simulink model "eVTOL_System"  (R2024b)
settings: Solver=FixedStepAuto  StartTime=0.0  StopTime=inf  RelTol=1e-3
undefined symbols (not defined in the file): airspeed, Battery, BCE12, BCE_Set_init, BMS_Controller_State, C, Cell10_P, Cell11_P, Cell12_P, Cell13_P, Cell14_P, Cell15_P, Cell16_P, Cell17_P, Cell18_P, Cell19_P, Cell1_N, Cell1_P, Cell20_P, Cell21_P, Cell22_P, Cell23_P, Cell24_P, Cell2_P, Cell3_P, Cell4_P, Cell5_P, Cell6_P, Cell7_P, Cell8_P, Cell9_P, Charging_State, CityMission, control, controlParams, ControlSampleTime, CriticalTiltAngle, currentFactor, CV_Gain, ddx, ddy, ddz, Device_01, Device_02, DiscIntNeverNeededParam, dx, dy, dz, Earth, env, F, F28379D_ADC_MaxCount, F28379D_ADC_Vmax, FixedWingMission, flightState, Foc_Ki_IxTcpu, Foc_Ki_S, Foc_Kp_I, Foc_Kp_S, fractalcoef ... (+68)
libraries: fl_lib x1115, nesl_utility x617, slrealtimeethercatlib x217, simulink x130, canmsglib x101, speedgoatlib_IO611_obsolete x91, slpidlib x49, mcbcontrolslib x44, slrealtimeutilitieslib x35, speedgoatlib_hdlCoder_IO3xx x31, dspstat3 x24, mcbpositiondecoderlib x12
(part 24 of 31)

== system eVTOL_System/Flight Controller/Guidance Test Bench/ControlType/Guidance Testbench/Guidance Logic/Guidance Stateflow/Guidance Mode Selector/GuidanceLogic.FIXED_WING_ORBIT.ORBIT ==
  ToWP : Inport
  States : Inport  Port=2
  Action Port : ActionPort
      settings: CopyFcn=Stateflow.SLINSF.SimulinkMan.removeBlockPreDeleteFcn  PreDeleteFcn=Stateflow.SLINSF.SimulinkMan.unsafePredeleteFcn
  Abs1 : Abs  SaturateOnIntegerOverflow=off
  Bus Creator : BusCreator  Inputs=5  OutDataTypeStr=Bus: AAC  NonVirtualBus=on
      settings: InheritFromInputs=off
  Bus Selector : BusSelector  OutputSignals=position,params
  Bus Selector1 : BusSelector  OutputSignals=Xe,course  OutputAsBus=on
  Bus to Vector : BusToVector
  Constant : Constant  Value=control.cruiseSpeed
  Constant1 : Constant  Value=0
  Data Type Conversion : DataTypeConversion  OutDataTypeStr=uint8  SaturateOnIntegerOverflow=off  RndMeth=Floor
  Lookahead Distance : Constant  Value=control.L1  OutDataTypeStr=double
  Relational Operator : RelationalOperator  Operator=>  OutDataTypeStr=boolean  RndMeth=Simplest  InputSameDT=off
  Selector : Selector  InputPortWidth=3  IndexOptions=Index vector (dialog)  Indices=3  OutputSizes=1
  Selector1 : Selector  InputPortWidth=4  IndexOptions=Index vector (dialog)  Indices=2  OutputSizes=1
  Selector2 : Selector  InputPortWidth=4  IndexOptions=Index vector (dialog)  Indices=1  OutputSizes=1
  Selector3 : Selector  InputPortWidth=4  IndexOptions=Index vector (dialog)  Indices=3  OutputSizes=1
  Terminator{,1..3} (4 alike) : Terminator
  UAV Orbit Follower : uavalgslib/Orbit Follower  UAVType=fixed-wing  MinOrbitRadius=control.turningRadius  MinLookaheadDistance=control.L1  ExternalReset=none  ShowCrossTrackErrorOutput=off  ShowNumTurnsOutput=on  SimulateUsing=Code generation
  Unary Minus : UnaryMinus
  Status : Outport
  aacSP : Outport  Port=2
  wires:
  Bus to Vector/1 -> UAV Orbit Follower/1
  Selector2/1 -> UAV Orbit Follower/3
  Bus Selector/1 -> UAV Orbit Follower/2, Selector/1  "<position>"
  ToWP/1 -> Bus Selector/1
  Bus Selector/2 -> Selector1/1, Selector3/1, Selector2/1  "<params>"
  Selector3/1 -> Relational Operator/2
  Relational Operator/1 -> Data Type Conversion/1
  UAV Orbit Follower/4 -> Terminator/1
  UAV Orbit Follower/5 -> Terminator1/1
  Bus Selector1/1 -> Bus to Vector/1
  States/1 -> Bus Selector1/1
  UAV Orbit Follower/1 -> Terminator2/1  "LAP"
  Lookahead Distance/1 -> UAV Orbit Follower/5, Bus Creator/4  "L1"
  Bus Creator/1 -> aacSP/1
  UAV Orbit Follower/2 -> Bus Creator/3  "course"
  Constant/1 -> Bus Creator/1  "airspeed"
  Unary Minus/1 -> Bus Creator/2  "altitude"
  UAV Orbit Follower/3 -> Terminator3/1  "YawCmd"
  Selector/1 -> Unary Minus/1
  UAV Orbit Follower/6 -> Abs1/1
  Abs1/1 -> Relational Operator/1
  Selector1/1 -> UAV Orbit Follower/4
  Constant1/1 -> Bus Creator/5  "climbrate"
  Data Type Conversion/1 -> Status/1

== system eVTOL_System/Flight Controller/Guidance Test Bench/ControlType/Guidance Testbench/Guidance Logic/Guidance Stateflow/Guidance Mode Selector/GuidanceLogic.FIXED_WING_WAYPOINT.WAYPOINT ==
  note: This subsystem selects a lookahead point on the path and provides a desired course. Desired course is later converted to desired lateral acceleration (and roll setpoint)
  States : Inport
  ToWP : Inport  Port=2
  FromWP : Inport  Port=3
  Action Port : ActionPort
      settings: CopyFcn=Stateflow.SLINSF.SimulinkMan.removeBlockPreDeleteFcn  PreDeleteFcn=Stateflow.SLINSF.SimulinkMan.unsafePredeleteFcn
  Bus Creator : BusCreator  Inputs=5  OutDataTypeStr=Bus: AAC  NonVirtualBus=on
      settings: InheritFromInputs=off
  Bus Selector : BusSelector  OutputSignals=Xe,course  OutputAsBus=on
  Bus Selector1 : BusSelector  OutputSignals=position
  Bus Selector2 : BusSelector  OutputSignals=position
  Bus to Vector : BusToVector
  Constant : Constant  Value=control.cruiseSpeed
  Constant1 : Constant  Value=0
  Data Type Conversion : DataTypeConversion  SaturateOnIntegerOverflow=off  RndMeth=Floor
  Lookahead Distance : Constant  Value=control.L1  OutDataTypeStr=double
  MATLAB Function : MATLAB Function  TreatAsAtomicUnit=on
  Scope : Scope
  Terminator : Terminator
  Terminator1 : Terminator
  Terminator2 : Terminator
  Waypoint Follower : uavalgslib/Waypoint Follower  UAVType=fixed-wing  StartFrom=first  TransitionRadiusSource=internal  TransitionRadius=FWControl.transitionRadius  MinLookaheadDistance=control.L1  HoverAtLastWaypoint=off  YawInput=off  ShowCrossTrackErrorOutput=off  ShowStatusOutput=on  SimulateUsing=Code generation
  Status : Outport
  aacSP : Outport  Port=2
  wires:
  Lookahead Distance/1 -> Waypoint Follower/3, Bus Creator/4  "L1"
  Waypoint Follower/1 -> Terminator/1  "LAP"
  Waypoint Follower/3 -> Terminator1/1  "YawCmd"
  Waypoint Follower/4 -> Terminator2/1
  Constant/1 -> Bus Creator/1  "airspeed"
  States/1 -> Bus Selector/1
  Bus Selector/1 -> Bus to Vector/1
  Waypoint Follower/5 -> Scope/1, Data Type Conversion/1
  Data Type Conversion/1 -> Status/1
  Bus Creator/1 -> aacSP/1
  MATLAB Function/1(wps) -> Waypoint Follower/2
  Bus to Vector/1 -> Waypoint Follower/1
  ToWP/1 -> Bus Selector1/1
  FromWP/1 -> Bus Selector2/1
  Bus Selector1/1 -> MATLAB Function/1(toWP)  "<position>"
  Bus Selector2/1 -> MATLAB Function/2(fromWP)  "<position>"
  MATLAB Function/2(alt) -> Bus Creator/2
  Waypoint Follower/2 -> Bus Creator/3  "course"
  Constant1/1 -> Bus Creator/5  "climbrate"

== system eVTOL_System/Flight Controller/Guidance Test Bench/ControlType/Guidance Testbench/Guidance Logic/Guidance Stateflow/Guidance Mode Selector/GuidanceLogic.ForwardTransition ==
  Action Port : ActionPort
      settings: CopyFcn=Stateflow.SLINSF.SimulinkMan.removeBlockPreDeleteFcn  PreDeleteFcn=Stateflow.SLINSF.SimulinkMan.unsafePredeleteFcn
  Bus Creator1 : BusCreator  Inputs=3  OutDataTypeStr=Bus: innerLoopCmdsBus  NonVirtualBus=on
  Constant : Constant  Value=0
  Constant1 : Constant  Value=0
  Constant2 : Constant  Value=0
  Constant3 : Constant  Value=[0 0 0]
  Data Type Conversion : DataTypeConversion  OutDataTypeStr=uint8  SaturateOnIntegerOverflow=off  RndMeth=Floor
  Status : Outport
  InnerLoopCmds : Outport  Port=2  OutDataTypeStr=Bus: innerLoopCmdsBus
  wires:
  Constant3/1 -> Bus Creator1/1  "LAP"
  Bus Creator1/1 -> InnerLoopCmds/1
  Constant1/1 -> Bus Creator1/2  "HeadingCmd"
  Constant2/1 -> Bus Creator1/3  "YawCmd"
  Data Type Conversion/1 -> Status/1
  Constant/1 -> Data Type Conversion/1

== system eVTOL_System/Flight Controller/Guidance Test Bench/ControlType/Guidance Testbench/Guidance Logic/Guidance Stateflow/Guidance Mode Selector/GuidanceLogic.Land.Descend ==
  ToWP : Inport
  Action Port : ActionPort
      settings: CopyFcn=Stateflow.SLINSF.SimulinkMan.removeBlockPreDeleteFcn  PreDeleteFcn=Stateflow.SLINSF.SimulinkMan.unsafePredeleteFcn
  Bus Creator : BusCreator  Inputs=3  OutDataTypeStr=Bus: innerLoopCmdsBus  NonVirtualBus=on
      settings: InheritFromInputs=off
  Bus Selector : BusSelector  OutputSignals=position,params
  Demux1 : Demux  Outputs=[2 1]
  Hdg Cmd Sat : Saturate  UpperLimit=pi  LowerLimit=-pi
      settings: AttributesFormatString=[%<UpperLimit> %<LowerLimit>]
  Mux : Mux  Inputs=2
  Selector1 : Selector  InputPortWidth=4  IndexOptions=Index vector (dialog)  Indices=4  OutputSizes=1
  Selector3 : Selector  InputPortWidth=4  IndexOptions=Index vector (dialog)  Indices=4  OutputSizes=1
  Yaw Cmd Sat : Saturate  UpperLimit=pi  LowerLimit=-pi
      settings: AttributesFormatString=[%<UpperLimit> %<LowerLimit>]
  InnerLoopCmds : Outport  OutDataTypeStr=Bus: innerLoopCmdsBus
  wires:
  Bus Creator/1 -> InnerLoopCmds/1
  Mux/1 -> Bus Creator/1  "LAP"
  Bus Selector/2 -> Selector1/1, Selector3/1  "<params>"
  Bus Selector/1 -> Demux1/1  "<position>"
  Yaw Cmd Sat/1 -> Bus Creator/3  "YawCmd"
  Hdg Cmd Sat/1 -> Bus Creator/2  "HeadingCmd"
  ToWP/1 -> Bus Selector/1
  Demux1/2 -> Mux/2
  Demux1/1 -> Mux/1
  Selector1/1 -> Yaw Cmd Sat/1
  Selector3/1 -> Hdg Cmd Sat/1

== system eVTOL_System/Flight Controller/Guidance Test Bench/ControlType/Guidance Testbench/Guidance Logic/Guidance Stateflow/Guidance Mode Selector/GuidanceLogic.Land.ToLand ==
  Pose : Inport
  ToWP : Inport  Port=2
  FromWP : Inport  Port=3
  Action Port : ActionPort
      settings: CopyFcn=Stateflow.SLINSF.SimulinkMan.removeBlockPreDeleteFcn  PreDeleteFcn=Stateflow.SLINSF.SimulinkMan.unsafePredeleteFcn
  Bus Creator1 : BusCreator  Inputs=3  OutDataTypeStr=Bus: innerLoopCmdsBus  NonVirtualBus=on
  Constant : Constant  Value=0  OutDataTypeStr=uint8
  Lookahead Distance : Constant  Value=15  OutDataTypeStr=double
  MATLAB Function : MATLAB Function  TreatAsAtomicUnit=on
  Scope : Scope
  Waypoint Follower : uavalgslib/Waypoint Follower  UAVType=multirotor  StartFrom=closest  TransitionRadiusSource=internal  TransitionRadius=10  MinLookaheadDistance=0.1  HoverAtLastWaypoint=off  YawInput=on  ShowCrossTrackErrorOutput=off  ShowStatusOutput=off  SimulateUsing=Code generation
  Status : Outport
  InnerLoopCmds : Outport  Port=2  OutDataTypeStr=Bus: innerLoopCmdsBus
  wires:
  Constant/1 -> Status/1
  MATLAB Function/1(wps) -> Waypoint Follower/2
  Lookahead Distance/1 -> Waypoint Follower/3
  Bus Creator1/1 -> InnerLoopCmds/1
  ToWP/1 -> MATLAB Function/2(ToWP)
  Waypoint Follower/2 -> Bus Creator1/2  "HeadingCmd"
  FromWP/1 -> MATLAB Function/1(FromWP)
  Waypoint Follower/4 -> Scope/1
  Waypoint Follower/3 -> Bus Creator1/3  "YawCmd"
  Pose/1 -> Waypoint Follower/1
  Waypoint Follower/1 -> Bus Creator1/1  "LAP"

== system eVTOL_System/Flight Controller/Guidance Test Bench/ControlType/Guidance Testbench/Guidance Logic/Guidance Stateflow/Guidance Mode Selector/GuidanceLogic.Land.WingsLevel ==
  Pose : Inport
  ToWP : Inport  Port=2
  FromWP : Inport  Port=3
  Action Port : ActionPort
      settings: CopyFcn=Stateflow.SLINSF.SimulinkMan.removeBlockPreDeleteFcn  PreDeleteFcn=Stateflow.SLINSF.SimulinkMan.unsafePredeleteFcn
  Bus Creator1 : BusCreator  Inputs=3  OutDataTypeStr=Bus: innerLoopCmdsBus  NonVirtualBus=on
  Constant : Constant  Value=0  OutDataTypeStr=uint8
  Constant1 : Constant  Value=0
  Constant2 : Constant  Value=0
  MATLAB Function : MATLAB Function  TreatAsAtomicUnit=on
  Terminator : Terminator
  Status : Outport
  InnerLoopCmds : Outport  Port=2  OutDataTypeStr=Bus: innerLoopCmdsBus
  wires:
  Bus Creator1/1 -> InnerLoopCmds/1
  Constant/1 -> Status/1
  MATLAB Function/1(outWPS) -> Bus Creator1/1  "LAP"
  Constant1/1 -> Bus Creator1/2  "HeadingCmd"
  FromWP/1 -> MATLAB Function/1(FromWP)
  Constant2/1 -> Bus Creator1/3  "YawCmd"
  ToWP/1 -> MATLAB Function/2(ToWP)
  Pose/1 -> Terminator/1

== system eVTOL_System/Flight Controller/Guidance Test Bench/ControlType/Guidance Testbench/Guidance Logic/Guidance Stateflow/Guidance Mode Selector/GuidanceLogic.Orbit ==
  ToWP : Inport
  Pose : Inport  Port=2
  Action Port : ActionPort
      settings: CopyFcn=Stateflow.SLINSF.SimulinkMan.removeBlockPreDeleteFcn  PreDeleteFcn=Stateflow.SLINSF.SimulinkMan.unsafePredeleteFcn
  Abs : Abs  SaturateOnIntegerOverflow=off
  Bus Creator : BusCreator  Inputs=3  OutDataTypeStr=Bus: innerLoopCmdsBus  NonVirtualBus=on
  Bus Selector : BusSelector  OutputSignals=position,params
  Data Type Conversion : DataTypeConversion  OutDataTypeStr=uint8  SaturateOnIntegerOverflow=off  RndMeth=Floor
  Lookahead Distance : Constant  Value=5  OutDataTypeStr=double
  Radius : Selector  InputPortWidth=4  IndexOptions=Index vector (dialog)  Indices=[3]  OutputSizes=1
  Relational Operator : RelationalOperator  Operator=>  OutDataTypeStr=boolean  RndMeth=Simplest  InputSameDT=off
  Sign : Signum  ZeroCross=off
  Terminator : Terminator
  Terminator1 : Terminator
  Turns : Selector  InputPortWidth=4  IndexOptions=Index vector (dialog)  Indices=[1]  OutputSizes=1
  UAV Orbit Follower : uavalgslib/Orbit Follower  UAVType=multirotor  MinOrbitRadius=1  MinLookaheadDistance=0.1  ExternalReset=none  ShowCrossTrackErrorOutput=off  ShowNumTurnsOutput=on  SimulateUsing=Code generation
  InnerLoopCmds : Outport  OutDataTypeStr=Bus: innerLoopCmdsBus
  Status : Outport  Port=2
  wires:
  Pose/1 -> UAV Orbit Follower/1
  Lookahead Distance/1 -> UAV Orbit Follower/5
  Abs/1 -> UAV Orbit Follower/3
  Bus Selector/1 -> UAV Orbit Follower/2  "<position>"
  ToWP/1 -> Bus Selector/1
  UAV Orbit Follower/1 -> Bus Creator/1  "LAP"
  Bus Creator/1 -> InnerLoopCmds/1
  UAV Orbit Follower/2 -> Bus Creator/2  "HeadingCmd"
  UAV Orbit Follower/3 -> Bus Creator/3  "YawCmd"
  Bus Selector/2 -> Turns/1, Radius/1  "<params>"
  Radius/1 -> Abs/1, Sign/1
  Sign/1 -> UAV Orbit Follower/4
  Relational Operator/1 -> Data Type Conversion/1
  Turns/1 -> Relational Operator/2
  Data Type Conversion/1 -> Status/1
  UAV Orbit Follower/6 -> Relational Operator/1
  UAV Orbit Follower/4 -> Terminator/1
  UAV Orbit Follower/5 -> Terminator1/1

== system eVTOL_System/Flight Controller/Guidance Test Bench/ControlType/Guidance Testbench/Guidance Logic/Guidance Stateflow/Guidance Mode Selector/GuidanceLogic.Takeoff ==
  ToWP : Inport
  Pose : Inport  Port=2
  Action Port : ActionPort
      settings: CopyFcn=Stateflow.SLINSF.SimulinkMan.removeBlockPreDeleteFcn  PreDeleteFcn=Stateflow.SLINSF.SimulinkMan.unsafePredeleteFcn
  Bus Creator : BusCreator  Inputs=3  OutDataTypeStr=Bus: innerLoopCmdsBus  NonVirtualBus=on
      settings: InheritFromInputs=off
  Bus Selector : BusSelector  OutputSignals=position,params
  Constant : Constant  Value=0  OutDataTypeStr=uint8
  Constant1 : Constant  Value=0
  Demux : Demux  Outputs=[2 2]
  Demux1 : Demux  Outputs=[2 1]
  Hdg. Cmd Sat : Saturate  UpperLimit=pi  LowerLimit=-pi
      settings: AttributesFormatString=[%<UpperLimit> %<LowerLimit>]
  Mux : Mux  Inputs=2
  Selector3 : Selector  InputPortWidth=4  IndexOptions=Index vector (dialog)  Indices=4  OutputSizes=1
  Terminator : Terminator
  Terminator1 : Terminator
  Yaw Cmd Sat : Saturate  UpperLimit=pi  LowerLimit=-pi
      settings: AttributesFormatString=[%<UpperLimit> %<LowerLimit>]
  InnerLoopCmds : Outport  OutDataTypeStr=Bus: innerLoopCmdsBus
  Status : Outport  Port=2
  wires:
  Hdg. Cmd Sat/1 -> Bus Creator/2  "HeadingCmd"
  Bus Creator/1 -> InnerLoopCmds/1
  Constant/1 -> Status/1
  Pose/1 -> Demux/1
  Yaw Cmd Sat/1 -> Bus Creator/3  "YawCmd"
  ToWP/1 -> Bus Selector/1
  Bus Selector/2 -> Selector3/1  "<params>"
  Mux/1 -> Bus Creator/1  "LAP"
  Demux/1 -> Mux/1
  Bus Selector/1 -> Demux1/1  "<position>"
  Demux/2 -> Terminator/1
  Demux1/1 -> Terminator1/1
  Selector3/1 -> Hdg. Cmd Sat/1
  Constant1/1 -> Yaw Cmd Sat/1
  Demux1/2 -> Mux/2

== system eVTOL_System/Flight Controller/Guidance Test Bench/ControlType/Guidance Testbench/Guidance Logic/Guidance Stateflow/Guidance Mode Selector/GuidanceLogic.WP ==
  FromWP : Inport
  Pose : Inport  Port=2
  ToWP : Inport  Port=3
  Action Port : ActionPort
      settings: CopyFcn=Stateflow.SLINSF.SimulinkMan.removeBlockPreDeleteFcn  PreDeleteFcn=Stateflow.SLINSF.SimulinkMan.unsafePredeleteFcn
  Back Transition Guard : Subsystem
  Bus Creator : BusCreator  Inputs=3  OutDataTypeStr=Bus: innerLoopCmdsBus  NonVirtualBus=on
  Constant : Constant  Value=0
  Data Type Conversion : DataTypeConversion  OutDataTypeStr=uint8  SaturateOnIntegerOverflow=off  RndMeth=Floor
  Dist2WP : Subsystem
  Lookahead Distance : Constant  Value=R_LOOKAHEAD  OutDataTypeStr=double
  MATLAB Function : MATLAB Function  TreatAsAtomicUnit=on
  Relational Operator : RelationalOperator  OutDataTypeStr=boolean  RndMeth=Simplest  InputSameDT=off
  Scope : Scope
  Terminator : Terminator
  Waypoint Follower : uavalgslib/Waypoint Follower  UAVType=multirotor  StartFrom=closest  TransitionRadiusSource=internal  TransitionRadius=R_WAYPOINTTRANSITION  MinLookaheadDistance=0.1  HoverAtLastWaypoint=off  YawInput=on  ShowCrossTrackErrorOutput=off  ShowStatusOutput=off  SimulateUsing=Code generation
  InnerLoopCmds : Outport  OutDataTypeStr=Bus: innerLoopCmdsBus
  Status : Outport  Port=2
  wires:
  Data Type Conversion/1 -> Status/1
  Bus Creator/1 -> InnerLoopCmds/1
  ToWP/1 -> Dist2WP/3(ToWP), MATLAB Function/2(ToWP)
  Waypoint Follower/1 -> Bus Creator/1  "LAP"
  MATLAB Function/1(wps) -> Waypoint Follower/2
  Waypoint Follower/2 -> Bus Creator/2  "HeadingCmd"
  Waypoint Follower/4 -> Scope/1
  Dist2WP/1(Dist) -> Relational Operator/2
  FromWP/1 -> Back Transition Guard/2(FromWP)
  Relational Operator/1 -> Data Type Conversion/1
  Back Transition Guard/1(PrevWP) -> Dist2WP/2(FromWP), MATLAB Function/1(FromWP)
  Pose/1 -> Back Transition Guard/1(Poses), Waypoint Follower/1, Dist2WP/1(Pose)
  Lookahead Distance/1 -> Relational Operator/1, Waypoint Follower/3
  Constant/1 -> Bus Creator/3  "YawCmd"
  Waypoint Follower/3 -> Terminator/1  "YawCmd"

== system eVTOL_System/Motor Drive/Controller/Controller_MIL/F28379D Firmware/Controller Algorithm/FOC/Current Control ==
  Iab : Inport
  Pos : Inport  Port=2
  Enable : Inport  Port=3
  Idq_ref_PU : Inport  Port=4
  SpeedRef : Inport  Port=5
  Kp_i : Inport  Port=6
  Ki_ixTcpu : Inport  Port=7
  Control_System : Subsystem
  ModWave : Outport  InitialOutput=0  VectorParamsAs1DForOutWhenUnconnected=off
  PWM_Enable : Outport  Port=2  InitialOutput=0  VectorParamsAs1DForOutWhenUnconnected=off
  wires:
  Idq_ref_PU/1 -> Control_System/4(Idq_ref_PU)  "Idq_ref"
  Pos/1 -> Control_System/2(Pos_PU)  "Pos_PU"
  Enable/1 -> Control_System/3(Enable)
  Iab/1 -> Control_System/1(Iab_meas_PU)  "Iab"
  SpeedRef/1 -> Control_System/5(SpeedRef)
  Control_System/1(ModWave) -> ModWave/1
  Control_System/2(PWM_Enable) -> PWM_Enable/1
  Kp_i/1 -> Control_System/6(Kp_i)
  Ki_ixTcpu/1 -> Control_System/7(Ki_ixTcpu)

== system eVTOL_System/Motor Drive/Controller/Controller_MIL/F28379D Firmware/Controller Algorithm/FOC/Speed Control MLD ==
  En_closedloop : Inport
  EnablePWM : Inport  Port=2
  SpeedRef : Inport  Port=3
  Speed_Meas_PU : Inport  Port=4
  Kp_S : Inport  Port=5
  Ki_S : Inport  Port=6
  AND : Logic  IconShape=distinctive  AllPortsSameDT=off  OutDataTypeStr=boolean
  Id_Ref : Constant  Value=0  OutDataTypeStr=single
  Mux : Mux  Inputs=2
  PI_Controller_Speed : Subsystem
  Speed_Ref_Selector : Subsystem
  IdqRef_PU : Outport  VectorParamsAs1DForOutWhenUnconnected=off
  wires:
  En_closedloop/1 -> PI_Controller_Speed/1(Enable), AND/1
  EnablePWM/1 -> AND/2
  SpeedRef/1 -> Speed_Ref_Selector/2(SpeedCommand)
  AND/1 -> Speed_Ref_Selector/1(Enable)
  Speed_Meas_PU/1 -> PI_Controller_Speed/3(N_fb), Speed_Ref_Selector/3(Speed_Ref_Open)
  Kp_S/1 -> PI_Controller_Speed/4(Kp_S)
  Speed_Ref_Selector/1(Speed_Ref_PU) -> PI_Controller_Speed/2(N_ref)
  Ki_S/1 -> PI_Controller_Speed/5(Ki_S)
  Id_Ref/1 -> Mux/1
  PI_Controller_Speed/1(Iq_ref) -> Mux/2
  Mux/1 -> IdqRef_PU/1

== system eVTOL_System/Motor Drive/Controller/Controller_MIL/F28379D Firmware/Controller Algorithm/Speed and Pos Decoder/IndexFinder ==
  In1 : Inport
  Enable : EnablePort
  AND : Logic  AllPortsSameDT=off  OutDataTypeStr=boolean
  Compare To Constant : simulink/Logic and Bit Operations/Compare To Constant  relop===  const=0  OutDataTypeStr=boolean
  Compare To Constant1 : simulink/Logic and Bit Operations/Compare To Constant  relop=>  const=0  OutDataTypeStr=boolean
  Delay3 : Delay  DelayLength=1
  IndexFound : Outport
  wires:
  In1/1 -> Delay3/1, Compare To Constant1/1
  Compare To Constant1/1 -> AND/2
  Compare To Constant/1 -> AND/1
  Delay3/1 -> Compare To Constant/1
  AND/1 -> IndexFound/1

== system eVTOL_System/Motor Drive/Controller1/Controller_MIL/F28379D Firmware/Controller Algorithm/FOC/Current Control ==
  Iab : Inport
  Pos : Inport  Port=2
  Enable : Inport  Port=3
  Idq_ref_PU : Inport  Port=4
  SpeedRef : Inport  Port=5
  Kp_i : Inport  Port=6
  Ki_ixTcpu : Inport  Port=7
  Control_System : Subsystem
  ModWave : Outport  InitialOutput=0  VectorParamsAs1DForOutWhenUnconnected=off
  PWM_Enable : Outport  Port=2  InitialOutput=0  VectorParamsAs1DForOutWhenUnconnected=off
  wires:
  Idq_ref_PU/1 -> Control_System/4(Idq_ref_PU)  "Idq_ref"
  Pos/1 -> Control_System/2(Pos_PU)  "Pos_PU"
  Enable/1 -> Control_System/3(Enable)
  Iab/1 -> Control_System/1(Iab_meas_PU)  "Iab"
  SpeedRef/1 -> Control_System/5(SpeedRef)
  Control_System/1(ModWave) -> ModWave/1
  Control_System/2(PWM_Enable) -> PWM_Enable/1
  Kp_i/1 -> Control_System/6(Kp_i)
  Ki_ixTcpu/1 -> Control_System/7(Ki_ixTcpu)

== system eVTOL_System/Motor Drive/Controller1/Controller_MIL/F28379D Firmware/Controller Algorithm/FOC/Speed Control MLD ==
  En_closedloop : Inport
  EnablePWM : Inport  Port=2
  SpeedRef : Inport  Port=3
  Speed_Meas_PU : Inport  Port=4
  Kp_S : Inport  Port=5
  Ki_S : Inport  Port=6
  AND : Logic  IconShape=distinctive  AllPortsSameDT=off  OutDataTypeStr=boolean
  Id_Ref : Constant  Value=0  OutDataTypeStr=single
  Mux : Mux  Inputs=2
  PI_Controller_Speed : Subsystem
  Speed_Ref_Selector : Subsystem
  IdqRef_PU : Outport  VectorParamsAs1DForOutWhenUnconnected=off
  wires:
  En_closedloop/1 -> PI_Controller_Speed/1(Enable), AND/1
  EnablePWM/1 -> AND/2
  SpeedRef/1 -> Speed_Ref_Selector/2(SpeedCommand)
  AND/1 -> Speed_Ref_Selector/1(Enable)
  Speed_Meas_PU/1 -> PI_Controller_Speed/3(N_fb), Speed_Ref_Selector/3(Speed_Ref_Open)
  Kp_S/1 -> PI_Controller_Speed/4(Kp_S)
  Speed_Ref_Selector/1(Speed_Ref_PU) -> PI_Controller_Speed/2(N_ref)
  Ki_S/1 -> PI_Controller_Speed/5(Ki_S)
  Id_Ref/1 -> Mux/1
  PI_Controller_Speed/1(Iq_ref) -> Mux/2
  Mux/1 -> IdqRef_PU/1

== system eVTOL_System/Motor Drive/Controller1/Controller_MIL/F28379D Firmware/Controller Algorithm/Speed and Pos Decoder/IndexFinder ==
  In1 : Inport
  Enable : EnablePort
  AND : Logic  AllPortsSameDT=off  OutDataTypeStr=boolean
  Compare To Constant : simulink/Logic and Bit Operations/Compare To Constant  relop===  const=0  OutDataTypeStr=boolean
  Compare To Constant1 : simulink/Logic and Bit Operations/Compare To Constant  relop=>  const=0  OutDataTypeStr=boolean
  Delay3 : Delay  DelayLength=1
  IndexFound : Outport
  wires:
  In1/1 -> Delay3/1, Compare To Constant1/1
  Compare To Constant1/1 -> AND/2
  Compare To Constant/1 -> AND/1
  Delay3/1 -> Compare To Constant/1
  AND/1 -> IndexFound/1

== system eVTOL_System/Motor Drive/Controller2/Controller_MIL/F28379D Firmware/Controller Algorithm/FOC/Current Control ==
  Iab : Inport
  Pos : Inport  Port=2
  Enable : Inport  Port=3
  Idq_ref_PU : Inport  Port=4
  SpeedRef : Inport  Port=5
  Kp_i : Inport  Port=6
  Ki_ixTcpu : Inport  Port=7
  Control_System : Subsystem
  ModWave : Outport  InitialOutput=0  VectorParamsAs1DForOutWhenUnconnected=off
  PWM_Enable : Outport  Port=2  InitialOutput=0  VectorParamsAs1DForOutWhenUnconnected=off
  wires:
  Idq_ref_PU/1 -> Control_System/4(Idq_ref_PU)  "Idq_ref"
  Pos/1 -> Control_System/2(Pos_PU)  "Pos_PU"
  Enable/1 -> Control_System/3(Enable)
  Iab/1 -> Control_System/1(Iab_meas_PU)  "Iab"
  SpeedRef/1 -> Control_System/5(SpeedRef)
  Control_System/1(ModWave) -> ModWave/1
  Control_System/2(PWM_Enable) -> PWM_Enable/1
  Kp_i/1 -> Control_System/6(Kp_i)
  Ki_ixTcpu/1 -> Control_System/7(Ki_ixTcpu)

== system eVTOL_System/Motor Drive/Controller2/Controller_MIL/F28379D Firmware/Controller Algorithm/FOC/Speed Control MLD ==
  En_closedloop : Inport
  EnablePWM : Inport  Port=2
  SpeedRef : Inport  Port=3
  Speed_Meas_PU : Inport  Port=4
  Kp_S : Inport  Port=5
  Ki_S : Inport  Port=6
  AND : Logic  IconShape=distinctive  AllPortsSameDT=off  OutDataTypeStr=boolean
  Id_Ref : Constant  Value=0  OutDataTypeStr=single
  Mux : Mux  Inputs=2
  PI_Controller_Speed : Subsystem
  Speed_Ref_Selector : Subsystem
  IdqRef_PU : Outport  VectorParamsAs1DForOutWhenUnconnected=off
  wires:
  En_closedloop/1 -> PI_Controller_Speed/1(Enable), AND/1
  EnablePWM/1 -> AND/2
  SpeedRef/1 -> Speed_Ref_Selector/2(SpeedCommand)
  AND/1 -> Speed_Ref_Selector/1(Enable)
  Speed_Meas_PU/1 -> PI_Controller_Speed/3(N_fb), Speed_Ref_Selector/3(Speed_Ref_Open)
  Kp_S/1 -> PI_Controller_Speed/4(Kp_S)
  Speed_Ref_Selector/1(Speed_Ref_PU) -> PI_Controller_Speed/2(N_ref)
  Ki_S/1 -> PI_Controller_Speed/5(Ki_S)
  Id_Ref/1 -> Mux/1
  PI_Controller_Speed/1(Iq_ref) -> Mux/2
  Mux/1 -> IdqRef_PU/1

== system eVTOL_System/Motor Drive/Controller2/Controller_MIL/F28379D Firmware/Controller Algorithm/Speed and Pos Decoder/IndexFinder ==
  In1 : Inport
  Enable : EnablePort
  AND : Logic  AllPortsSameDT=off  OutDataTypeStr=boolean
  Compare To Constant : simulink/Logic and Bit Operations/Compare To Constant  relop===  const=0  OutDataTypeStr=boolean
  Compare To Constant1 : simulink/Logic and Bit Operations/Compare To Constant  relop=>  const=0  OutDataTypeStr=boolean
  Delay3 : Delay  DelayLength=1
  IndexFound : Outport
  wires:
  In1/1 -> Delay3/1, Compare To Constant1/1
  Compare To Constant1/1 -> AND/2
  Compare To Constant/1 -> AND/1
  Delay3/1 -> Compare To Constant/1
  AND/1 -> IndexFound/1

== system eVTOL_System/Motor Drive/Controller3/Controller_MIL/F28379D Firmware/Controller Algorithm/FOC/Current Control ==
  Iab : Inport
  Pos : Inport  Port=2
  Enable : Inport  Port=3
  Idq_ref_PU : Inport  Port=4
  SpeedRef : Inport  Port=5
  Kp_i : Inport  Port=6
  Ki_ixTcpu : Inport  Port=7
  Control_System : Subsystem
  ModWave : Outport  InitialOutput=0  VectorParamsAs1DForOutWhenUnconnected=off
  PWM_Enable : Outport  Port=2  InitialOutput=0  VectorParamsAs1DForOutWhenUnconnected=off
  wires:
  Idq_ref_PU/1 -> Control_System/4(Idq_ref_PU)  "Idq_ref"
  Pos/1 -> Control_System/2(Pos_PU)  "Pos_PU"
  Enable/1 -> Control_System/3(Enable)
  Iab/1 -> Control_System/1(Iab_meas_PU)  "Iab"
  SpeedRef/1 -> Control_System/5(SpeedRef)
  Control_System/1(ModWave) -> ModWave/1
  Control_System/2(PWM_Enable) -> PWM_Enable/1
  Kp_i/1 -> Control_System/6(Kp_i)
  Ki_ixTcpu/1 -> Control_System/7(Ki_ixTcpu)

== system eVTOL_System/Motor Drive/Controller3/Controller_MIL/F28379D Firmware/Controller Algorithm/FOC/Speed Control MLD ==
  En_closedloop : Inport
  EnablePWM : Inport  Port=2
  SpeedRef : Inport  Port=3
  Speed_Meas_PU : Inport  Port=4
  Kp_S : Inport  Port=5
  Ki_S : Inport  Port=6
  AND : Logic  IconShape=distinctive  AllPortsSameDT=off  OutDataTypeStr=boolean
  Id_Ref : Constant  Value=0  OutDataTypeStr=single
  Mux : Mux  Inputs=2
  PI_Controller_Speed : Subsystem
  Speed_Ref_Selector : Subsystem
  IdqRef_PU : Outport  VectorParamsAs1DForOutWhenUnconnected=off
  wires:
  En_closedloop/1 -> PI_Controller_Speed/1(Enable), AND/1
  EnablePWM/1 -> AND/2
  SpeedRef/1 -> Speed_Ref_Selector/2(SpeedCommand)
  AND/1 -> Speed_Ref_Selector/1(Enable)
  Speed_Meas_PU/1 -> PI_Controller_Speed/3(N_fb), Speed_Ref_Selector/3(Speed_Ref_Open)
  Kp_S/1 -> PI_Controller_Speed/4(Kp_S)
  Speed_Ref_Selector/1(Speed_Ref_PU) -> PI_Controller_Speed/2(N_ref)
  Ki_S/1 -> PI_Controller_Speed/5(Ki_S)
  Id_Ref/1 -> Mux/1
  PI_Controller_Speed/1(Iq_ref) -> Mux/2
  Mux/1 -> IdqRef_PU/1

== system eVTOL_System/Motor Drive/Controller3/Controller_MIL/F28379D Firmware/Controller Algorithm/Speed and Pos Decoder/IndexFinder ==
  In1 : Inport
  Enable : EnablePort
  AND : Logic  AllPortsSameDT=off  OutDataTypeStr=boolean
  Compare To Constant : simulink/Logic and Bit Operations/Compare To Constant  relop===  const=0  OutDataTypeStr=boolean
  Compare To Constant1 : simulink/Logic and Bit Operations/Compare To Constant  relop=>  const=0  OutDataTypeStr=boolean
  Delay3 : Delay  DelayLength=1
  IndexFound : Outport
  wires:
  In1/1 -> Delay3/1, Compare To Constant1/1
  Compare To Constant1/1 -> AND/2
  Compare To Constant/1 -> AND/1
  Delay3/1 -> Compare To Constant/1
  AND/1 -> IndexFound/1

== system eVTOL_System/Battery System/Battery/HW Interface/BCE - HIL/Battery Cell Emulator/BCE Read /Subsystem/BCE Read  ==
  note: Cell 7
  note: Cell 2
  note: Cell 6
  note: Cell 8
  note: Cell 12
  note: Cell 11
  note: Cell 3
  note: Cell 5
  note: Cell 4
  note: Cell 10
  note: Cell 9
  note: Cell 1
  Bus Creator : BusCreator  Inputs=12  OutDataTypeStr=Bus: BCE_Get
      settings: InheritFromInputs=off
  Bus Creator{1..10,13..14} (12 alike) : BusCreator  Inputs=4  OutDataTypeStr=Bus: Cell_Get
      settings: InheritFromInputs=off
  Byte Packing{,1..9,12..13} (12 alike) : slrealtimeutilitieslib/Byte Packing  MaskPackedDataType=uint64  MaskUnpackedDataTypes={'uint32','uint32'}  MaskAlignment=1
  EtherCAT PDO Receive01 : slrealtimeethercatlib/EtherCAT PDO Receive  Priority=2  sig_name=Device_01 (BCE12-0505).Tx_Cell_01.voltage  sig_offset=16  sig_type=single  type_size=32  sig_dim=1  device_id=0  sample_time=0.001000
  EtherCAT PDO Receive02 : slrealtimeethercatlib/EtherCAT PDO Receive  Priority=2  sig_name=Device_01 (BCE12-0505).Tx_Cell_01.current  sig_offset=48  sig_type=single  type_size=32  sig_dim=1  device_id=0  sample_time=0.001000
  EtherCAT PDO Receive03 : slrealtimeethercatlib/EtherCAT PDO Receive  Priority=2  sig_name=Device_01 (BCE12-0505).Tx_Cell_01.chargeMSB  sig_offset=80  sig_type=uint32  type_size=32  sig_dim=1  device_id=0  sample_time=0.001000
  EtherCAT PDO Receive04 : slrealtimeethercatlib/EtherCAT PDO Receive  Priority=2  sig_name=Device_01 (BCE12-0505).Tx_Cell_01.chargeLSB  sig_offset=112  sig_type=uint32  type_size=32  sig_dim=1  device_id=0  sample_time=0.001000
  EtherCAT PDO Receive05 : slrealtimeethercatlib/EtherCAT PDO Receive  Priority=2  sig_name=Device_01 (BCE12-0505).Tx_Cell_02.voltage  sig_offset=160  sig_type=single  type_size=32  sig_dim=1  device_id=0  sample_time=0.001000
  EtherCAT PDO Receive06 : slrealtimeethercatlib/EtherCAT PDO Receive  Priority=2  sig_name=Device_01 (BCE12-0505).Tx_Cell_02.current  sig_offset=192  sig_type=single  type_size=32  sig_dim=1  device_id=0  sample_time=0.001000
  EtherCAT PDO Receive07 : slrealtimeethercatlib/EtherCAT PDO Receive  Priority=2  sig_name=Device_01 (BCE12-0505).Tx_Cell_02.chargeMSB  sig_offset=224  sig_type=uint32  type_size=32  sig_dim=1  device_id=0  sample_time=0.001000
  EtherCAT PDO Receive08 : slrealtimeethercatlib/EtherCAT PDO Receive  Priority=2  sig_name=Device_01 (BCE12-0505).Tx_Cell_02.chargeLSB  sig_offset=256  sig_type=uint32  type_size=32  sig_dim=1  device_id=0  sample_time=0.001000
  EtherCAT PDO Receive1 : slrealtimeethercatlib/EtherCAT PDO Receive  Priority=2  sig_name=Device_01 (BCE12-0505).Tx_Cell_01.status  sig_offset=0  sig_type=uint16  type_size=16  sig_dim=1  device_id=0  sample_time=0.001000
  EtherCAT PDO Receive10 : slrealtimeethercatlib/EtherCAT PDO Receive  Priority=2  sig_name=Device_01 (BCE12-0505).Tx_Cell_05.chargeMSB  sig_offset=656  sig_type=uint32  type_size=32  sig_dim=1  device_id=0  sample_time=0.001000
  EtherCAT PDO Receive11 : slrealtimeethercatlib/EtherCAT PDO Receive  Priority=2  sig_name=Device_01 (BCE12-0505).Tx_Cell_05.chargeLSB  sig_offset=688  sig_type=uint32  type_size=32  sig_dim=1  device_id=0  sample_time=0.001000
  EtherCAT PDO Receive12 : slrealtimeethercatlib/EtherCAT PDO Receive  Priority=2  sig_name=Device_01 (BCE12-0505).Tx_Cell_05.status  sig_offset=576  sig_type=uint16  type_size=16  sig_dim=1  device_id=0  sample_time=0.001000
  EtherCAT PDO Receive13 : slrealtimeethercatlib/EtherCAT PDO Receive  Priority=2  sig_name=Device_01 (BCE12-0505).Tx_Cell_06.chargeMSB  sig_offset=800  sig_type=uint32  type_size=32  sig_dim=1  device_id=0  sample_time=0.001000
  EtherCAT PDO Receive14 : slrealtimeethercatlib/EtherCAT PDO Receive  Priority=2  sig_name=Device_01 (BCE12-0505).Tx_Cell_06.chargeLSB  sig_offset=832  sig_type=uint32  type_size=32  sig_dim=1  device_id=0  sample_time=0.001000
  EtherCAT PDO Receive15 : slrealtimeethercatlib/EtherCAT PDO Receive  Priority=2  sig_name=Device_01 (BCE12-0505).Tx_Cell_06.status  sig_offset=720  sig_type=uint16  type_size=16  sig_dim=1  device_id=0  sample_time=0.001000
  EtherCAT PDO Receive16 : slrealtimeethercatlib/EtherCAT PDO Receive  Priority=2  sig_name=Device_01 (BCE12-0505).Tx_Cell_06.voltage  sig_offset=736  sig_type=single  type_size=32  sig_dim=1  device_id=0  sample_time=0.001000
  EtherCAT PDO Receive17 : slrealtimeethercatlib/EtherCAT PDO Receive  Priority=2  sig_name=Device_01 (BCE12-0505).Tx_Cell_06.current  sig_offset=768  sig_type=single  type_size=32  sig_dim=1  device_id=0  sample_time=0.001000
  EtherCAT PDO Receive18 : slrealtimeethercatlib/EtherCAT PDO Receive  Priority=2  sig_name=Device_01 (BCE12-0505).Tx_Cell_07.chargeMSB  sig_offset=944  sig_type=uint32  type_size=32  sig_dim=1  device_id=0  sample_time=0.001000
  EtherCAT PDO Receive19 : slrealtimeethercatlib/EtherCAT PDO Receive  Priority=2  sig_name=Device_01 (BCE12-0505).Tx_Cell_07.chargeLSB  sig_offset=976  sig_type=uint32  type_size=32  sig_dim=1  device_id=0  sample_time=0.001000
  EtherCAT PDO Receive2 : slrealtimeethercatlib/EtherCAT PDO Receive  Priority=2  sig_name=Device_01 (BCE12-0505).Tx_Cell_02.status  sig_offset=144  sig_type=uint16  type_size=16  sig_dim=1  device_id=0  sample_time=0.001000
  EtherCAT PDO Receive20 : slrealtimeethercatlib/EtherCAT PDO Receive  Priority=2  sig_name=Device_01 (BCE12-0505).Tx_Cell_07.status  sig_offset=864  sig_type=uint16  type_size=16  sig_dim=1  device_id=0  sample_time=0.001000
  EtherCAT PDO Receive21 : slrealtimeethercatlib/EtherCAT PDO Receive  Priority=2  sig_name=Device_01 (BCE12-0505).Tx_Cell_07.voltage  sig_offset=880  sig_type=single  type_size=32  sig_dim=1  device_id=0  sample_time=0.001000
  EtherCAT PDO Receive22 : slrealtimeethercatlib/EtherCAT PDO Receive  Priority=2  sig_name=Device_01 (BCE12-0505).Tx_Cell_07.current  sig_offset=912  sig_type=single  type_size=32  sig_dim=1  device_id=0  sample_time=0.001000
  EtherCAT PDO Receive23 : slrealtimeethercatlib/EtherCAT PDO Receive  Priority=2  sig_name=Device_01 (BCE12-0505).Tx_Cell_08.chargeMSB  sig_offset=1088  sig_type=uint32  type_size=32  sig_dim=1  device_id=0  sample_time=0.001000
  EtherCAT PDO Receive24 : slrealtimeethercatlib/EtherCAT PDO Receive  Priority=2  sig_name=Device_01 (BCE12-0505).Tx_Cell_08.chargeLSB  sig_offset=1120  sig_type=uint32  type_size=32  sig_dim=1  device_id=0  sample_time=0.001000
  EtherCAT PDO Receive25 : slrealtimeethercatlib/EtherCAT PDO Receive  Priority=2  sig_name=Device_01 (BCE12-0505).Tx_Cell_08.status  sig_offset=1008  sig_type=uint16  type_size=16  sig_dim=1  device_id=0  sample_time=0.001000
  EtherCAT PDO Receive26 : slrealtimeethercatlib/EtherCAT PDO Receive  Priority=2  sig_name=Device_01 (BCE12-0505).Tx_Cell_08.voltage  sig_offset=1024  sig_type=single  type_size=32  sig_dim=1  device_id=0  sample_time=0.001000
  EtherCAT PDO Receive27 : slrealtimeethercatlib/EtherCAT PDO Receive  Priority=2  sig_name=Device_01 (BCE12-0505).Tx_Cell_08.current  sig_offset=1056  sig_type=single  type_size=32  sig_dim=1  device_id=0  sample_time=0.001000
  EtherCAT PDO Receive28 : slrealtimeethercatlib/EtherCAT PDO Receive  Priority=2  sig_name=Device_01 (BCE12-0505).Tx_Cell_09.chargeMSB  sig_offset=1232  sig_type=uint32  type_size=32  sig_dim=1  device_id=0  sample_time=0.001000
  EtherCAT PDO Receive29 : slrealtimeethercatlib/EtherCAT PDO Receive  Priority=2  sig_name=Device_01 (BCE12-0505).Tx_Cell_09.chargeLSB  sig_offset=1264  sig_type=uint32  type_size=32  sig_dim=1  device_id=0  sample_time=0.001000
  EtherCAT PDO Receive3 : slrealtimeethercatlib/EtherCAT PDO Receive  Priority=2  sig_name=Device_01 (BCE12-0505).Tx_Cell_03.voltage  sig_offset=304  sig_type=single  type_size=32  sig_dim=1  device_id=0  sample_time=0.001000
  EtherCAT PDO Receive30 : slrealtimeethercatlib/EtherCAT PDO Receive  Priority=2  sig_name=Device_01 (BCE12-0505).Tx_Cell_09.status  sig_offset=1152  sig_type=uint16  type_size=16  sig_dim=1  device_id=0  sample_time=0.001000
  EtherCAT PDO Receive31 : slrealtimeethercatlib/EtherCAT PDO Receive  Priority=2  sig_name=Device_01 (BCE12-0505).Tx_Cell_09.voltage  sig_offset=1168  sig_type=single  type_size=32  sig_dim=1  device_id=0  sample_time=0.001000
  EtherCAT PDO Receive32 : slrealtimeethercatlib/EtherCAT PDO Receive  Priority=2  sig_name=Device_01 (BCE12-0505).Tx_Cell_09.current  sig_offset=1200  sig_type=single  type_size=32  sig_dim=1  device_id=0  sample_time=0.001000
  EtherCAT PDO Receive33 : slrealtimeethercatlib/EtherCAT PDO Receive  Priority=2  sig_name=Device_01 (BCE12-0505).Tx_Cell_10.chargeMSB  sig_offset=1376  sig_type=uint32  type_size=32  sig_dim=1  device_id=0  sample_time=0.001000
  EtherCAT PDO Receive34 : slrealtimeethercatlib/EtherCAT PDO Receive  Priority=2  sig_name=Device_01 (BCE12-0505).Tx_Cell_10.chargeLSB  sig_offset=1408  sig_type=uint32  type_size=32  sig_dim=1  device_id=0  sample_time=0.001000
  EtherCAT PDO Receive35 : slrealtimeethercatlib/EtherCAT PDO Receive  Priority=2  sig_name=Device_01 (BCE12-0505).Tx_Cell_10.status  sig_offset=1296  sig_type=uint16  type_size=16  sig_dim=1  device_id=0  sample_time=0.001000
  EtherCAT PDO Receive36 : slrealtimeethercatlib/EtherCAT PDO Receive  Priority=2  sig_name=Device_01 (BCE12-0505).Tx_Cell_10.voltage  sig_offset=1312  sig_type=single  type_size=32  sig_dim=1  device_id=0  sample_time=0.001000
  EtherCAT PDO Receive37 : slrealtimeethercatlib/EtherCAT PDO Receive  Priority=2  sig_name=Device_01 (BCE12-0505).Tx_Cell_10.current  sig_offset=1344  sig_type=single  type_size=32  sig_dim=1  device_id=0  sample_time=0.001000
  EtherCAT PDO Receive38 : slrealtimeethercatlib/EtherCAT PDO Receive  Priority=2  sig_name=Device_01 (BCE12-0505).Tx_Cell_11.chargeMSB  sig_offset=1520  sig_type=uint32  type_size=32  sig_dim=1  device_id=0  sample_time=0.001000
  EtherCAT PDO Receive39 : slrealtimeethercatlib/EtherCAT PDO Receive  Priority=2  sig_name=Device_01 (BCE12-0505).Tx_Cell_11.chargeLSB  sig_offset=1552  sig_type=uint32  type_size=32  sig_dim=1  device_id=0  sample_time=0.001000
  EtherCAT PDO Receive4 : slrealtimeethercatlib/EtherCAT PDO Receive  Priority=2  sig_name=Device_01 (BCE12-0505).Tx_Cell_03.current  sig_offset=336  sig_type=single  type_size=32  sig_dim=1  device_id=0  sample_time=0.001000
  EtherCAT PDO Receive40 : slrealtimeethercatlib/EtherCAT PDO Receive  Priority=2  sig_name=Device_01 (BCE12-0505).Tx_Cell_11.status  sig_offset=1440  sig_type=uint16  type_size=16  sig_dim=1  device_id=0  sample_time=0.001000
  EtherCAT PDO Receive41 : slrealtimeethercatlib/EtherCAT PDO Receive  Priority=2  sig_name=Device_01 (BCE12-0505).Tx_Cell_11.voltage  sig_offset=1456  sig_type=single  type_size=32  sig_dim=1  device_id=0  sample_time=0.001000
  EtherCAT PDO Receive42 : slrealtimeethercatlib/EtherCAT PDO Receive  Priority=2  sig_name=Device_01 (BCE12-0505).Tx_Cell_11.current  sig_offset=1488  sig_type=single  type_size=32  sig_dim=1  device_id=0  sample_time=0.001000
  EtherCAT PDO Receive43 : slrealtimeethercatlib/EtherCAT PDO Receive  Priority=2  sig_name=Device_01 (BCE12-0505).Tx_Cell_12.chargeMSB  sig_offset=1664  sig_type=uint32  type_size=32  sig_dim=1  device_id=0  sample_time=0.001000
  EtherCAT PDO Receive44 : slrealtimeethercatlib/EtherCAT PDO Receive  Priority=2  sig_name=Device_01 (BCE12-0505).Tx_Cell_12.chargeLSB  sig_offset=1696  sig_type=uint32  type_size=32  sig_dim=1  device_id=0  sample_time=0.001000
  EtherCAT PDO Receive45 : slrealtimeethercatlib/EtherCAT PDO Receive  Priority=2  sig_name=Device_01 (BCE12-0505).Tx_Cell_12.status  sig_offset=1584  sig_type=uint16  type_size=16  sig_dim=1  device_id=0  sample_time=0.001000
  EtherCAT PDO Receive46 : slrealtimeethercatlib/EtherCAT PDO Receive  Priority=2  sig_name=Device_01 (BCE12-0505).Tx_Cell_12.voltage  sig_offset=1600  sig_type=single  type_size=32  sig_dim=1  device_id=0  sample_time=0.001000
  EtherCAT PDO Receive47 : slrealtimeethercatlib/EtherCAT PDO Receive  Priority=2  sig_name=Device_01 (BCE12-0505).Tx_Cell_12.current  sig_offset=1632  sig_type=single  type_size=32  sig_dim=1  device_id=0  sample_time=0.001000
  EtherCAT PDO Receive49 : slrealtimeethercatlib/EtherCAT PDO Receive  Priority=2  sig_name=Device_01 (BCE12-0505).Tx_Cell_04.chargeMSB  sig_offset=512  sig_type=uint32  type_size=32  sig_dim=1  device_id=0  sample_time=0.001000
  EtherCAT PDO Receive5 : slrealtimeethercatlib/EtherCAT PDO Receive  Priority=2  sig_name=Device_01 (BCE12-0505).Tx_Cell_03.chargeMSB  sig_offset=368  sig_type=uint32  type_size=32  sig_dim=1  device_id=0  sample_time=0.001000
  EtherCAT PDO Receive50 : slrealtimeethercatlib/EtherCAT PDO Receive  Priority=2  sig_name=Device_01 (BCE12-0505).Tx_Cell_04.chargeLSB  sig_offset=544  sig_type=uint32  type_size=32  sig_dim=1  device_id=0  sample_time=0.001000
  EtherCAT PDO Receive51 : slrealtimeethercatlib/EtherCAT PDO Receive  Priority=2  sig_name=Device_01 (BCE12-0505).Tx_Cell_04.status  sig_offset=432  sig_type=uint16  type_size=16  sig_dim=1  device_id=0  sample_time=0.001000
  EtherCAT PDO Receive52 : slrealtimeethercatlib/EtherCAT PDO Receive  Priority=2  sig_name=Device_01 (BCE12-0505).Tx_Cell_05.voltage  sig_offset=592  sig_type=single  type_size=32  sig_dim=1  device_id=0  sample_time=0.001000
  EtherCAT PDO Receive53 : slrealtimeethercatlib/EtherCAT PDO Receive  Priority=2  sig_name=Device_01 (BCE12-0505).Tx_Cell_05.current  sig_offset=624  sig_type=single  type_size=32  sig_dim=1  device_id=0  sample_time=0.001000
  EtherCAT PDO Receive6 : slrealtimeethercatlib/EtherCAT PDO Receive  Priority=2  sig_name=Device_01 (BCE12-0505).Tx_Cell_03.chargeLSB  sig_offset=400  sig_type=uint32  type_size=32  sig_dim=1  device_id=0  sample_time=0.001000
  EtherCAT PDO Receive7 : slrealtimeethercatlib/EtherCAT PDO Receive  Priority=2  sig_name=Device_01 (BCE12-0505).Tx_Cell_03.status  sig_offset=288  sig_type=uint16  type_size=16  sig_dim=1  device_id=0  sample_time=0.001000
  EtherCAT PDO Receive8 : slrealtimeethercatlib/EtherCAT PDO Receive  Priority=2  sig_name=Device_01 (BCE12-0505).Tx_Cell_04.voltage  sig_offset=448  sig_type=single  type_size=32  sig_dim=1  device_id=0  sample_time=0.001000
  EtherCAT PDO Receive9 : slrealtimeethercatlib/EtherCAT PDO Receive  Priority=2  sig_name=Device_01 (BCE12-0505).Tx_Cell_04.current  sig_offset=480  sig_type=single  type_size=32  sig_dim=1  device_id=0  sample_time=0.001000
  Data : Outport  OutDataTypeStr=Bus: BCE_Get
  wires:
  EtherCAT PDO Receive04/1 -> Byte Packing/2
  EtherCAT PDO Receive53/1 -> Bus Creator3/3  "Cell5_current"
  Bus Creator7/1 -> Bus Creator/9  "Cell09"
  EtherCAT PDO Receive1/1 -> Bus Creator1/1  "Cell1_status"
  EtherCAT PDO Receive40/1 -> Bus Creator9/1  "Cell11_status"
  EtherCAT PDO Receive39/1 -> Byte Packing8/2
  EtherCAT PDO Receive18/1 -> Byte Packing4/1
  Byte Packing13/1 -> Bus Creator14/4  "Cell4_charge"
  Bus Creator14/1 -> Bus Creator/4  "Cell04"
  EtherCAT PDO Receive21/1 -> Bus Creator5/2  "Cell7_voltage"
  EtherCAT PDO Receive52/1 -> Bus Creator3/2  "Cell5_voltage"
  EtherCAT PDO Receive15/1 -> Bus Creator4/1  "Cell6_status"
  EtherCAT PDO Receive11/1 -> Byte Packing2/2
  EtherCAT PDO Receive26/1 -> Bus Creator6/2  "Cell8_voltage"
  EtherCAT PDO Receive33/1 -> Byte Packing7/1
  EtherCAT PDO Receive12/1 -> Bus Creator3/1  "Cell5_status"
  Byte Packing2/1 -> Bus Creator3/4  "Cell5_charge"
  Byte Packing4/1 -> Bus Creator5/4  "Cell7_charge"
  Byte Packing6/1 -> Bus Creator7/4  "Cell9_charge"
  EtherCAT PDO Receive7/1 -> Bus Creator13/1  "Cell3_status"
  Bus Creator4/1 -> Bus Creator/6  "Cell06"
  Bus Creator6/1 -> Bus Creator/8  "Cell08"
  EtherCAT PDO Receive30/1 -> Bus Creator7/1  "Cell9_status"
  EtherCAT PDO Receive4/1 -> Bus Creator13/3  "Cell3_current"
  Bus Creator13/1 -> Bus Creator/3  "Cell03"
  Byte Packing7/1 -> Bus Creator8/4  "Cell10_charge"
  EtherCAT PDO Receive01/1 -> Bus Creator1/2  "Cell1_voltage"
  EtherCAT PDO Receive35/1 -> Bus Creator8/1  "Cell10_status"
  EtherCAT PDO Receive29/1 -> Byte Packing6/2
  EtherCAT PDO Receive27/1 -> Bus Creator6/3  "Cell8_current"
  EtherCAT PDO Receive32/1 -> Bus Creator7/3  "Cell9_current"
  EtherCAT PDO Receive41/1 -> Bus Creator9/2  "Cell11_voltage"
  EtherCAT PDO Receive5/1 -> Byte Packing12/1
  EtherCAT PDO Receive3/1 -> Bus Creator13/2  "Cell3_voltage"
  EtherCAT PDO Receive46/1 -> Bus Creator10/2  "Cell12_voltage"
  EtherCAT PDO Receive6/1 -> Byte Packing12/2
  EtherCAT PDO Receive17/1 -> Bus Creator4/3  "Cell6_current"
  EtherCAT PDO Receive9/1 -> Bus Creator14/3  "Cell4_current"
  Bus Creator9/1 -> Bus Creator/11  "Cell11"
  EtherCAT PDO Receive43/1 -> Byte Packing9/1
  EtherCAT PDO Receive44/1 -> Byte Packing9/2
  EtherCAT PDO Receive45/1 -> Bus Creator10/1  "Cell12_status"
  EtherCAT PDO Receive23/1 -> Byte Packing5/1
  EtherCAT PDO Receive37/1 -> Bus Creator8/3  "Cell10_current"
  EtherCAT PDO Receive8/1 -> Bus Creator14/2  "Cell4_voltage"
  EtherCAT PDO Receive14/1 -> Byte Packing3/2
  EtherCAT PDO Receive49/1 -> Byte Packing13/1
  EtherCAT PDO Receive19/1 -> Byte Packing4/2
  EtherCAT PDO Receive24/1 -> Byte Packing5/2
  Bus Creator2/1 -> Bus Creator/2  "Cell02"
  Bus Creator5/1 -> Bus Creator/7  "Cell07"
  Byte Packing8/1 -> Bus Creator9/4  "Cell11_charge"
  Byte Packing1/1 -> Bus Creator2/4  "Cell2_charge"
  Bus Creator10/1 -> Bus Creator/12  "Cell12"
  Bus Creator8/1 -> Bus Creator/10  "Cell10"
  EtherCAT PDO Receive28/1 -> Byte Packing6/1
  Byte Packing3/1 -> Bus Creator4/4  "Cell6_charge"
  EtherCAT PDO Receive13/1 -> Byte Packing3/1
  EtherCAT PDO Receive16/1 -> Bus Creator4/2  "Cell6_voltage"
  EtherCAT PDO Receive51/1 -> Bus Creator14/1  "Cell4_status"
  EtherCAT PDO Receive05/1 -> Bus Creator2/2  "Cell2_voltage"
  EtherCAT PDO Receive06/1 -> Bus Creator2/3  "Cell2_current"
  EtherCAT PDO Receive25/1 -> Bus Creator6/1  "Cell8_status"
  EtherCAT PDO Receive31/1 -> Bus Creator7/2  "Cell9_voltage"
  Byte Packing12/1 -> Bus Creator13/4  "Cell3_charge"
  Byte Packing/1 -> Bus Creator1/4  "Cell1_charge"
  EtherCAT PDO Receive38/1 -> Byte Packing8/1
  EtherCAT PDO Receive50/1 -> Byte Packing13/2
  Bus Creator3/1 -> Bus Creator/5  "Cell05"
  EtherCAT PDO Receive22/1 -> Bus Creator5/3  "Cell7_current"
  Byte Packing9/1 -> Bus Creator10/4  "Cell12_charge"
  Byte Packing5/1 -> Bus Creator6/4  "Cell8_charge"
  Bus Creator1/1 -> Bus Creator/1  "Cell01"
  EtherCAT PDO Receive36/1 -> Bus Creator8/2  "Cell10_voltage"
  EtherCAT PDO Receive07/1 -> Byte Packing1/1
  EtherCAT PDO Receive47/1 -> Bus Creator10/3  "Cell12_current"
  EtherCAT PDO Receive10/1 -> Byte Packing2/1
  EtherCAT PDO Receive20/1 -> Bus Creator5/1  "Cell7_status"
  EtherCAT PDO Receive42/1 -> Bus Creator9/3  "Cell11_current"
  EtherCAT PDO Receive02/1 -> Bus Creator1/3  "Cell1_current"
  EtherCAT PDO Receive34/1 -> Byte Packing7/2
  EtherCAT PDO Receive2/1 -> Bus Creator2/1  "Cell2_status"
  Bus Creator/1 -> Data/1
  EtherCAT PDO Receive03/1 -> Byte Packing/1
  EtherCAT PDO Receive08/1 -> Byte Packing1/2
